simulink model "UnitDelay3Model"  (R2018b)
settings: Solver=FixedStepAuto  StartTime=0.0  StopTime=3.0  FixedStep=0.5  RelTol=1e-3
settings Model: Creator=Reichl  LastModifiedBy=Reichl
settings DataIOCC: FinalStateName=xFinalStates3  SaveFinalState=on  SaveFormat=Array  SaveState=on  StateSaveName=xStates3  TimeSaveName=tout3  OutputSaveName=yout3
settings SFSimCC: SimUseLocalCustomCode=off
settings RTWCC: RTWUseLocalCustomCode=off
settings CodeAppCC: StateflowObjectComments=on

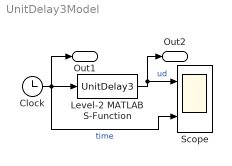
== system UnitDelay3Model ==
  Clock : Clock
  Level-2 MATLAB S-Function : M-S-Function  FunctionName=UnitDelay3  Parameters=-3, -2, -1
  Scope : Scope  NumInputPorts=2
  Out1 : Outport
  Out2 : Outport  Port=2
  wires:
  Clock/1 -> Scope/2, Out1/1, Level-2 MATLAB S-Function/1  "time"
  Level-2 MATLAB S-Function/1 -> Out2/1, Scope/1  "ud"
